simulink library "monroe_library"  (R2012b)
settings: Solver=ode45  StartTime=0.0  StopTime=10.0  RelTol=1e-3
values from neighbouring files (symbols this model uses):
  input_bit_width = ', num2str(input_bit_width))    [fft_direct_draw.m]
undefined symbols (not defined in the file or in its folder): gcbh, xlBlockLoadCallback
libraries: xbsIndex_r4 x1880, monroe_library x159, casper_library x13, xps_library x1
(part 19 of 43)

== system monroe_library/direct_coeff_gen/coeff_gen_stage_2_group_2 ==
  sync : Inport
  Concat : xbsIndex_r4/Concat  num_inputs=2  dbl_ovrd=off  block_type=concat
  Concat1 : xbsIndex_r4/Concat  num_inputs=2  dbl_ovrd=off  block_type=concat
  Concat2 : xbsIndex_r4/Concat  num_inputs=2  dbl_ovrd=off  block_type=concat
  Constant : xbsIndex_r4/Constant  arith_type=Boolean  const=0  n_bits=16  bin_pt=14  explicit_period=on  period=1  equ=P=C  opselect=C  inp2=PCIN>>17  opr=+  inp1=P  carry=CIN  dbl_ovrd=off  block_type=constant
  Constant1 : xbsIndex_r4/Constant  arith_type=Boolean  const=1  n_bits=16  bin_pt=14  explicit_period=off  period=1  equ=P=C  opselect=C  inp2=PCIN>>17  opr=+  inp1=P  carry=CIN  dbl_ovrd=off  block_type=constant
  Constant3 : xbsIndex_r4/Constant  arith_type=Signed (2's comp)  const=0  n_bits=18  bin_pt=17  explicit_period=on  period=1  equ=P=C  opselect=C  inp2=PCIN>>17  opr=+  inp1=P  carry=CIN  dbl_ovrd=off  block_type=constant
  Constant4 : xbsIndex_r4/Constant  arith_type=Boolean  const=0  n_bits=16  bin_pt=14  explicit_period=off  period=1  equ=P=C  opselect=C  inp2=PCIN>>17  opr=+  inp1=P  carry=CIN  dbl_ovrd=off  block_type=constant
  Constant5 : xbsIndex_r4/Constant  arith_type=Unsigned  const=2  n_bits=10  bin_pt=0  explicit_period=on  period=1  equ=P=C  opselect=C  inp2=PCIN>>17  opr=+  inp1=P  carry=CIN  dbl_ovrd=off  block_type=constant
  Counter : xbsIndex_r4/Counter  cnt_type=Free Running  cnt_to=Inf  operation=Up  start_count=0  cnt_by_val=1  arith_type=Unsigned  n_bits=10  bin_pt=0  load_pin=on  rst=off  en=off  explicit_period=on  period=1  dbl_ovrd=off  use_behavioral_HDL=off  implementation=Fabric  block_type=counter
  Delay : xbsIndex_r4/Delay  en=off  latency=0  dbl_ovrd=off  reg_retiming=off  block_type=delay
  Dual Port RAM4 : xbsIndex_r4/Dual Port RAM  depth=2048  initVector=[0 -0.00153398018628477 -0.00306795676296598 -0.00460192612044857 -0.00613588464915448 -0.0076698287395311 -0.00920375478205982 -0.0107376591672645 -0.0122715382857199 -0.0138053885280604 -0.0153392062849881 -0.0168729879472817 -0.0184067299058048 -0.0199404285515144 -0.0214740802754695 -0.0230076814688394 -0.0245412285229123 -0.0260747178291039 -0.0276081457789657 -0.0291415087641937 -0.0306748031766366 -0.0322080254083046 -0.0337411718513776 -0.0352742388982139 -0.0368072229413588 -0.0383401203735527 -0.0398729275877398 -0.0414056409770767 -0.0429382569349408 -0.0444707718549387 -0.0460031821309146 -0.0475354841569593 -0.049067674327418 -0.0505997490368993 -0.0521317046802833 -0.0536635376527305 -0.0551952443496899 -0.0567268211669077 -0.0582582645004358 -0.0597895707466399 -0.0613207363022086 -0.0628517575641614 -0.0643826309298575 -0.0659133527970038 -0.0674439195636641 -0.0689743276282667 -0.0705045733896139 -0.0720346532468893 -0.0735645635996674 -0.0750943008479213 -0.0766238613920315 -0.0781532416327942 -0.0796824379714301 -0.0812114468095924 -0.0827402645493757 -0.0842688875933241 -0.0857973123444399 -0.0873255352061921 -0.0888535525825246 -0.090381360877865 -0.0919089564971327 -0.0934363358457478 -0.094963495329639 -0.0964904313552526 -0.0980171403295606 -0.0995436186600693 -0.101069862754828 -0.102595869022436 -0.104121633872055 -0.105647153713411 -0.107172424956809 -0.108697444013139 -0.110222207293883 -0.111746711211127 -0.113270952177564 -0.11479492660651 -0.116318630911905 -0.117842061508325 -0.119365214810991 -0.120888087235777 -0.122410675199216 -0.123932975118512 -0.125454983411546 -0.126976696496886 -0.128498110793793 -0.130019222722233 -0.131540028702883 -0.133060525157139 -0.134580708507126 -0.136100575175706 -0.137620121586486 -0.139139344163826 -0.140658239332849 -0.142176803519448 -0.143695033150294 -0.145212924652847 -0.146730474455362 -0.148247678986896 -0.149764534677322 -0.15128103795733 -0.152797185258443 -0.15431297301302 -0.155828397654265 -0.157343455616238 -0.158858143333861 -0.160372457242928 -0.161886393780112 -0.163399949382973 -0.16491312048997 -0.166425903540464 -0.167938294974731 -0.169450291233968 -0.170961888760301 -0.172473083996796 -0.173983873387464 -0.175494253377271 -0.177004220412149 -0.178513770938998 -0.1800229014057 -0.181531608261125 -0.183039887955141 -0.18454773693862 -0.186055151663447 -0.18756212858253 -0.189068664149806 -0.190574754820253 -0.192080397049892 -0.193585587295804 -0.195090322016128 -0.19659459767008 -0.198098410717954 -0.199601757621131 -0.201104634842092 -0.202607038844421 -0.204108966092817 -0.205610413053099 -0.207111376192219 -0.208611851978263 -0.21011183688047 -0.211611327369228 -0.213110319916091 -0.214608810993787 -0.21610679707622 -0.217604274638484 -0.21910124015687 -0.220597690108874 -0.222093620973204 -0.22358902922979 -0.225083911359793 -0.22657826384561 -0.228072083170886 -0.229565365820519 -0.231058108280671 -0.232550307038775 -0.234041958583543 -0.235533059404975 -0.237023605994367 -0.238513594844318 -0.240003022448741 -0.241491885302869 -0.242980179903264 -0.244467902747824 -0.245955050335795 -0.247441619167773 -0.24892760574572 -0.250413006572965 -0.251897818154217 -0.25338203699557 -0.254865659604515 -0.256348682489943 -0.257831102162159 -0.259312915132886 -0.260794117915276 -0.262274707023914 -0.263754678974831 -0.265234030285512 -0.266712757474898 -0.268190857063403 -0.269668325572915 -0.271145159526808 -0.272621355449949 -0.274096909868706 -0.275571819310958 -0.2770460803061 -0.278519689385053 -0.279992643080273 -0.281464937925758 -0.282936570457055 -0.284407537211272 -0.285877834727081 -0.28734745954473 -0.288816408206049 -0.290284677254462 -0.291752263234989 -0.293219162694259 -0.294685372180514 -0.296150888243624 -0.297615707435086 -0.29907982630804 -0.300543241417273 -0.302005949319228 -0.303467946572011 -0.304929229735402 -0.306389795370861 -0.307849640041535 -0.309308760312269 -0.310767152749611 -0.312224813921825 ...(+33767 chars)]  distributed_mem=Block RAM  init_a=0  init_b=0  rst_a=off  rst_b=off  en_a=off  en_b=off  latency=2  write_mode_A=No Read On Write  write_mode_B=No Read On Write  dbl_ovrd=off  optimize=Area  use_rpm=on  block_type=dpram
  Reinterpret : xbsIndex_r4/Reinterpret  force_arith_type=on  arith_type=Unsigned  force_bin_pt=on  bin_pt=0  block_type=reinterpret
      settings: infoedit="Changes signal type without altering the binary representation.   You can changed the signal between signed and unsigned, and relocate the binary point.<br><br>Hardware notes: In hardware this block costs nothing.<br><br>Example:  Suppose the input is 6 bits wide, signed, with 2 fractional bits, and the output is forced to unsigned with 0 fractional bits.  Then an input of -2.0 (1110.00 in binary 2's complement) becomes an output of 56 (111000 in binary)."
  Reinterpret1 : xbsIndex_r4/Reinterpret  force_arith_type=on  arith_type=Unsigned  force_bin_pt=on  bin_pt=0  block_type=reinterpret
      settings: infoedit="Changes signal type without altering the binary representation.   You can changed the signal between signed and unsigned, and relocate the binary point.<br><br>Hardware notes: In hardware this block costs nothing.<br><br>Example:  Suppose the input is 6 bits wide, signed, with 2 fractional bits, and the output is forced to unsigned with 0 fractional bits.  Then an input of -2.0 (1110.00 in binary 2's complement) becomes an output of 56 (111000 in binary)."
  count_slice : xbsIndex_r4/Slice  nbits=10  boolean_output=off  mode=Upper Bit Location + Width  bit1=0  base1=MSB of Input  bit0=0  base0=MSB of Input  dbl_ovrd=off  block_type=slice
  coeff : Outport
  wires:
  count_slice/1 -> Concat1/2, Concat/2  "xlsub2_Counter_out1"
  Constant3/1 -> Dual Port RAM4/5, Dual Port RAM4/2  "xlsub2_Constant3_out1"
  Constant/1 -> Dual Port RAM4/6, Dual Port RAM4/3  "xlsub2_Constant_out1"
  Reinterpret1/1 -> Concat2/2  "xlsub2_Reinterpret1_out1"
  Dual Port RAM4/2 -> Reinterpret1/1  "xlsub2_Dual_Port_RAM4_out2"
  Reinterpret/1 -> Concat2/1  "xlsub2_Reinterpret_out1"
  Dual Port RAM4/1 -> Reinterpret/1  "xlsub2_Dual_Port_RAM4_out1"
  Concat1/1 -> Dual Port RAM4/4  "xlsub2_Concat1_out1"
  Concat/1 -> Dual Port RAM4/1  "xlsub2_Concat_out1"
  Delay/1 -> coeff/1
  Concat2/1 -> Delay/1  "xlsub2_Concat2_out1"
  Counter/1 -> count_slice/1
  Constant5/1 -> Counter/2  "xlsub2_Constant5_out1"
  sync/1 -> Counter/1
  Constant4/1 -> Concat1/1  "xlsub2_Constant4_out1"
  Constant1/1 -> Concat/1  "xlsub2_Constant1_out1"
